simulink model "FSM_Jacob2"  (R2025b)
settings: Solver=VariableStepAuto  StartTime=0.0  StopTime=10.0  RelTol=1e-3
settings Model: Creator=jacob  LastModifiedBy=jacob

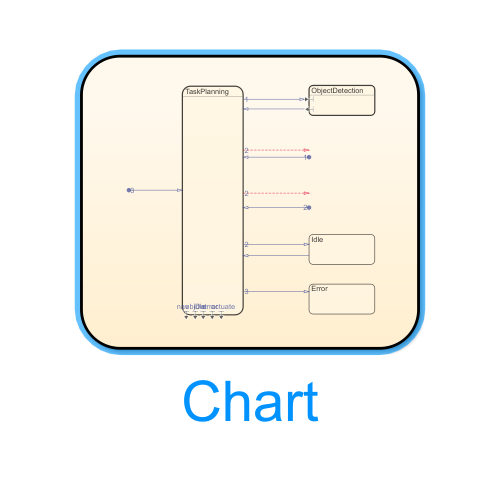
[thumbnail: Simulink's stored preview of the top-level diagram]
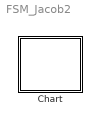
== system FSM_Jacob2 ==
  Chart : Stateflow chart  TreatAsAtomicUnit=on

== stateflow chart FSM_Jacob2/Chart ==
  state planTasks
    state updateOrderProgress
    updateOrderProgress -> (junction 422)
    (junction 422) -> 393 [order 1] : [orderComplete]{obj=='face'}
    389 -> updateOrderProgress
    (junction 422) -> (junction 424) [order 2]
    (junction 426) -> 393
    (junction 424) -> (junction 426) : {obj==burgerOrder(k)}
    (junction 396) -> (junction 426)
    391 -> (junction 396) : {obj=='stopSign'}
    (junction 395) -> (junction 396)
    324 -> (junction 395) : {obj='ingredients'}
    (junction 339) -> (junction 395)
    332 -> (junction 334)
    (junction 334) -> (junction 339) [order 1] : [obj=='ingredients']{obj=burgerOrder(1)}
    (junction 334) -> (junction 337) [order 2]
    (junction 355) -> (junction 339)
    (junction 337) -> (junction 355) [order 1] : [obj=='face']{obj=='customer'}
    (junction 337) -> (junction 343) [order 2]
    (junction 343) -> 371 [order 1] : [obj=='burgerBun']{grasperTask=='pickup'}
    (junction 343) -> (junction 349) [order 2]
    (junction 347) -> 371
    (junction 349) -> (junction 347) [order 1] : [obj=='burgerPatty']{grasperTask=='pickup'}
    (junction 349) -> (junction 353) [order 2]
    (junction 386) -> (junction 347)
    (junction 353) -> (junction 386) [order 1] : [obj=='customer']{grasperTask=='deposit'}
    (junction 353) -> (junction 357) [order 2]
    (junction 357) -> 322 [order 1] : [obj=='trafficLight']
    (junction 357) -> (junction 361) [order 2]
    (junction 361) -> 367 : [obj=='stopSign']
  state goToObj
    state analyzeCam
    state scan
    state GNC
    234 -> goToObj.analyzeCam
    goToObj.analyzeCam -> (junction 228)
    (junction 228) -> (junction 189)
    (junction 189) -> (junction 203) [order 1] : [arrived]
    (junction 203) -> 237 [order 1] : [inView]
    (junction 226) -> (junction 228)
    (junction 189) -> (junction 195) [order 2]
    (junction 203) -> (junction 206) [order 2]
    (junction 206) -> scan : [~inView]
    scan -> (junction 429)
    (junction 429) -> (junction 221) [order 1] : [~scanTimeout]
    (junction 429) -> (junction 431) [order 2]
    (junction 221) -> (junction 219)
    (junction 431) -> 433
    (junction 195) -> (junction 215) [order 1] : [inView]{targetCoord=estimation}
    (junction 215) -> GNC
    GNC -> (junction 219)
    (junction 195) -> (junction 199) [order 2]
    (junction 216) -> (junction 215)
    (junction 219) -> (junction 224)
    (junction 199) -> (junction 216) : [~inView]{targetCoord=aPriori}
    (junction 224) -> (junction 226)
  state taskAborted
  state waitForGreen
    state detectColor
    257 -> (junction 439)
    detectColor -> (junction 263)
    (junction 263) -> 273 [order 1] : [color=='green']
    (junction 439) -> detectColor
    (junction 438) -> (junction 439)
    (junction 263) -> (junction 278) [order 2]
    (junction 278) -> (junction 438) [order 1] : [color=='red']
    (junction 278) -> 275 [order 2]
  state useGrasper
    state getIntoPosition
      state analyzeCam
      state maneuver
      useGrasper.getIntoPosition.analyzeCam -> (junction 282)
      (junction 282) -> 298 [order 1] : [inPosition]
      290 -> (junction 293)
      (junction 293) -> useGrasper.getIntoPosition.analyzeCam
      (junction 282) -> (junction 286) [order 2]
      (junction 295) -> (junction 293)
      maneuver -> (junction 295)
      (junction 286) -> maneuver
    state pickup
    state deposit
    402 -> 291
    299 -> (junction 373)
    (junction 373) -> pickup [order 2] : [grasperTask=='pickup']
    pickup -> 407
    (junction 373) -> (junction 375) [order 1]
    (junction 375) -> deposit [order 1] : [grasperTask=='deposit']
    deposit -> 410
    (junction 375) -> 413 [order 2]
  state taskComplete
  327 -> 235
  434 -> (junction 309)
  (junction 309) -> taskAborted
  (junction 307) -> (junction 309)
  238 -> 333
  323 -> 258
  274 -> 325
  276 -> (junction 307)
  (junction 305) -> (junction 307)
  372 -> 403
  408 -> 390
  414 -> (junction 305)
  411 -> 392
  368 -> taskComplete
